simulink model "mf"  (R2021b)
settings: Solver=VariableStepAuto  StartTime=0.0  StopTime=6  RelTol=1e-3
settings Model: Creator=Dear Fatemeh  LastModifiedBy=Mahban
settings SolverCC: AlgebraicLoopSolver=TrustRegion
settings DataIOCC: ReturnWorkspaceOutputs=off
settings DebuggingCC: SFMachineParentedDataDiag=warning  ArithmeticOperatorsInVariantConditions=warning
settings SFSimCC: CustomCodeUndefinedFunction=UseInterfaceOnly

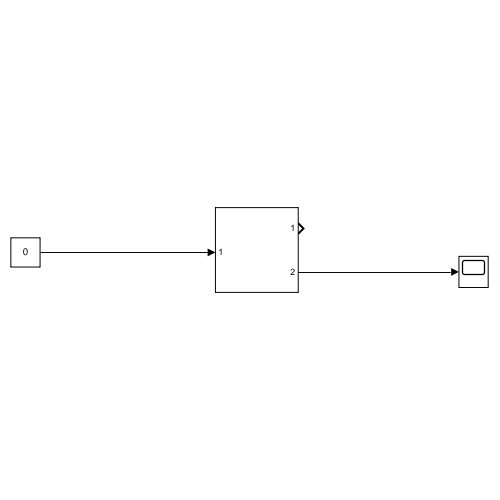
[thumbnail: Simulink's stored preview of the top-level diagram]
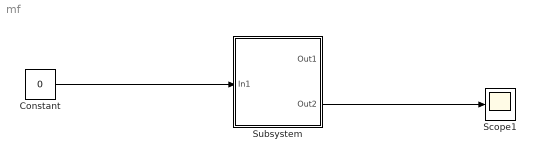
== system mf ==
  Constant : Constant  Value=0
  Scope1 : Scope
  Subsystem : Subsystem
  wires:
  Constant/1 -> Subsystem/1(In1)
  Subsystem/2(Out2) -> Scope1/1

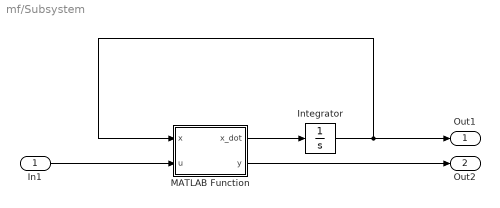
== system mf/Subsystem ==
  In1 : Inport
  Integrator : Integrator  InitialCondition=rand(6,1)
  MATLAB Function : MATLAB Function  TreatAsAtomicUnit=on
  Out1 : Outport  VectorParamsAs1DForOutWhenUnconnected=off
  Out2 : Outport  Port=2  VectorParamsAs1DForOutWhenUnconnected=off
  wires:
  In1/1 -> MATLAB Function/2(u)
  MATLAB Function/1(x_dot) -> Integrator/1
  Integrator/1 -> Out1/1, MATLAB Function/1(x)
  MATLAB Function/2(y) -> Out2/1

== matlab function mf/Subsystem/MATLAB Function ==
  data: x input; u input; x_dot output; y output
function [x_dot,y]  = fcn(x,u)
m1 = 2
m2 = 0.1
m3 = 0.1
r1 = 0.1
r2 = 0.1
g = 9.8

x1 = x(1)
x2 = x(2)
x3 = x(3)
x4 = x(4)
x5 = x(5)
x6 = x(6)

a = m2+m3
b = cos(x3)*cos(x5)
c = sin(x3-x5)
d = m2*a*sin(x3)^2 + m1*m3*c^2 + m1*m2
e = 2*m2^2 + m1*m3 + 2*m2*m3 + 2*m1*m2 + m1*m3*cos(2*x5)
f = m2*a*sin(2*x3) - m1*m3*sin(2*(x5-x3))
h = m2*m3*sin(x3)*cos(x5) + m1*m3*c

Q=(m2*g*a*sin(x3)*cos(x3))/(-d*x3)
W=m2*r1*a*x4*sin(x3)/d
R=m2*m3*r2*x6*(sin(x5-2*x3)-sin(x5))/(-2*d)
T=g*e*sin(x3)/(2*r1*d*x3)
Y=f*x4/(-2*d)
U=m1*m3*g*b*sin(x5)/(-r1*d*x5)
I=r2*h*x6/(-r1*d)
O=m1*g*a*b*sin(x3)/(-r2*d*x3)
P=m1*r1*a*c*x4/(r2*d)
S=m1*g*a*((cos(x3))^2)*sin(x5)/(r2*d*x5)
D=m1*m3*x6*sin(2*(x5-x3))/(-2*d)
A = [0 1 0 0 0 0;0 0 Q W 0 R;0 0 0 1 0 0;0 0 T Y U I;0 0 0 0 0 1;0 0 O P S D] 
B = [0 (m2+m3*c^2)/d 0 (m2*cos(x3)-m3*c*sin(x5))/(-r1*d) 0 (m2*cos(x3)-m3*c*sin(x5))/(-r1*d)]'
C = [0 0 1 0 0 0;0 0 0 0 1 0]
K = [18.7422 13.1195 -340.2858 -10.4880 387.3212 26.8517]
x_dot = (A-B*K)*x
y = C*x
end
